simulink model "test_zynq_zcu216"  (R2018b)
settings: Solver=VariableStepAuto  StartTime=0.0  StopTime=10.0  RelTol=1e-3
undefined symbols (not defined in the file): es1
libraries: xbsIndex_r4 x19
settings Model: Creator=mcb  LastModifiedBy=mcb

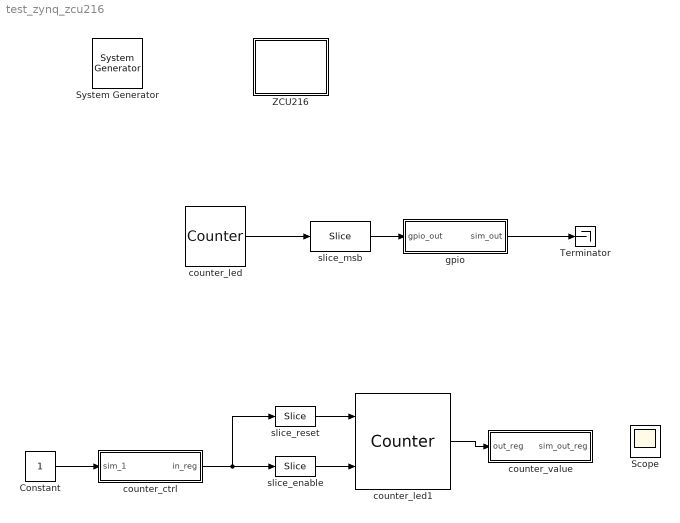
== system test_zynq_zcu216 ==
  " System Generator" : xbsIndex_r4/ System Generator  Tag=genX  xilinxfamily=zynquplusRFSOCes1  part=xczu49dr  speed=-2-e-es1  package=ffvf1760  synthesis_tool=XST  clock_wrapper=Clock Enables  directory=/home/mcb/git/casper-astro/mlib_devel/jasper_library/test_models/test_zynq_zcu216/sysgen  proj_type=Vivado  Synth_file=Vivado Synthesis Defaults  Impl_file=Vivado Implementation Defaults  testbench=off  simulink_period=1  sysclk_period=10  dcm_input_clock_period=10  incr_netlist=off  trim_vbits=Everywhere in SubSystem  dbl_ovrd=According to Block Masks  core_generation=According to Block Masks  run_coregen=off  deprecated_control=off  eval_field=0  block_type=sysgen
  Constant : Constant
  Scope : Scope
  Terminator : Terminator
  ZCU216 : Subsystem  Tag=xps:xsg  mask(xsg core config){hw_sys=ZCU216:xczu49dr, clk_src=adc_clk, clk_rate=100, sample_period=1, synthesis_tool=XST}
      mask prompts: hw_sys "Hardware Platform"; clk_src "User IP Clock source"; clk_rate "User IP Clock Rate (MHz)"; sample_period "Sample Period"; synthesis_tool "Synthesis Tool:"
      mask help:
      | The XSG Core Config block is used to configure the System Generator design
      | for the casper_xps toolflow. Settings here are used to configure the
      | Xilinx System Generator block parameters automatically, and control toolflow
      | script  execution. It needs to be at the top level of all designs being compiled
      | with the casper_xps toolflow.
      mask init:
      | xps_xsg_zcu216_conf_mask;
      mask Help: eval('xlWeb([getenv(''MLIB_ROOT''), ''\doc\html\sys_xsg_core_config\sys_xsg_core_config.html''])')
      mask TypeOptions hw_sys: ZCU216:xczu49dr
      mask TypeOptions clk_src: sys_clk | adc_clk
      mask TypeOptions synthesis_tool: Leonardo Spectrum | Synplify | Synplify Pro | XST
      mask Display: fprintf(['ZCU216']);
  counter_ctrl : Subsystem  Tag=xps:sw_reg  AncestorBlock=xps_library/Memory/software_register  mask(swreg){io_dir=From Processor, io_delay=0, init_val=0, sample_period=1, names=reg, bitwidths=32, bin_pts=0, arith_types=0, sim_port=on, show_format=off}
      mask prompts: io_dir "I/O direction"; io_delay "I/O delay"; init_val "Initial Value"; sample_period "Sample period"; names "Bitfield names [msb...lsb]"; bitwidths "Bitfield widths"; bin_pts "Bitfield binary pts"; arith_types "Bitfield types, ufix=0, fix=1, bool=2"; sim_port "Provide sim input/output?"; show_format "Print format string?"
      mask help: A 32-bit software-accessible register. Can be divided into bitfields of varying widths and types using the fields in the block mask.
      mask init:
      | swreg_init(gcb)
      settings: AttributesFormatString=1input
      mask TypeOptions io_dir: To Processor | From Processor
      mask Callback io_dir:
      | mask_enables = get_param(gcb, 'MaskEnables');
      | mask_names = get_param(gcb, 'MaskNames');
      | if strcmp(get_param(gcb, 'io_dir'), 'To Processor'),
      |     mask_enables{ismember(mask_names, 'sample_period')} = 'off';
      | else
      |     mask_enables{ismember(mask_names, 'sample_period')} = 'on';
      | end
      | set_param(gcb, 'MaskEnables', mask_enables);
      mask DialogControl ParameterTabVar0 Prompt: Setup
  counter_led : xbsIndex_r4/Counter  cnt_type=Free Running  cnt_to=Inf  operation=Up  start_count=0  cnt_by_val=1  arith_type=Unsigned  n_bits=28  bin_pt=0  load_pin=off  rst=off  en=off  explicit_period=on  period=1  use_behavioral_HDL=off  implementation=Fabric  dbl_ovrd=off  block_type=counter
  counter_led1 : xbsIndex_r4/Counter  cnt_type=Free Running  cnt_to=Inf  operation=Up  start_count=0  cnt_by_val=1  arith_type=Unsigned  n_bits=32  bin_pt=0  load_pin=off  rst=on  en=on  explicit_period=on  period=1  use_behavioral_HDL=off  implementation=Fabric  dbl_ovrd=off  block_type=counter
  counter_value : Subsystem  Tag=xps:sw_reg  AncestorBlock=xps_library/Memory/software_register  mask(swreg){io_dir=To Processor, io_delay=0, init_val=0, sample_period=1, names=reg, bitwidths=32, bin_pts=0, arith_types=0, sim_port=on, show_format=off}
      mask prompts: io_dir "I/O direction"; io_delay "I/O delay"; init_val "Initial Value"; sample_period "Sample period"; names "Bitfield names [msb...lsb]"; bitwidths "Bitfield widths"; bin_pts "Bitfield binary pts"; arith_types "Bitfield types, ufix=0, fix=1, bool=2"; sim_port "Provide sim input/output?"; show_format "Print format string?"
      mask help: A 32-bit software-accessible register. Can be divided into bitfields of varying widths and types using the fields in the block mask.
      mask init:
      | swreg_init(gcb)
      settings: AttributesFormatString=1output
      mask TypeOptions io_dir: To Processor | From Processor
      mask Callback io_dir:
      | mask_enables = get_param(gcb, 'MaskEnables');
      | mask_names = get_param(gcb, 'MaskNames');
      | if strcmp(get_param(gcb, 'io_dir'), 'To Processor'),
      |     mask_enables{ismember(mask_names, 'sample_period')} = 'off';
      | else
      |     mask_enables{ismember(mask_names, 'sample_period')} = 'on';
      | end
      | set_param(gcb, 'MaskEnables', mask_enables);
      mask DialogControl ParameterTabVar0 Prompt: Setup
  gpio : Subsystem  Tag=xps:gpio  AncestorBlock=xps_library/IO/gpio  mask(gpio){io_group_params_forwarded=on, io_group=ROACH2:led, io_group_real=led, io_group_custom=0, io_dir=out, arith_type=Boolean, bitwidth=1, bin_pt=0, bit_index=0, sample_period=1, use_single_ended=off, use_ddr=off, reg_iob=on, reg_clk_phase=0, termination=None}
      mask prompts: io_group_params_forwarded "Have the io_group params been forwarded yet?"; io_group "I/O group"; io_group_real "I/O group"; io_group_custom "Custom I/O group"; io_dir "I/O direction"; arith_type "Data Type"; bitwidth "Data bitwidth"; bin_pt "Data binary point"; bit_index "GPIO bit index"; sample_period "Sample period"; use_single_ended "Use as single-ended"; use_ddr "Use DDR"; reg_iob "Pack register in the pad"; reg_clk_phase "Register clock phase"; termination "Termination method"
      mask help:
      | GPIO interfaces for CASPER hardware.
      |
      | For usage of LEDs on SKARAB boards, please note that the board will boot into 'BSP mode' by default. To change the control of the Front Panel LEDs to your design, execute the command 'control_front_panel_leds_write()' on your SKARAB CASPERFPGA object via the transport layer.
      |
      | For more information please click help below.
      mask init:
      | gpio_mask;
      mask Help: If you've come here for more help, unfortunately I'm going to direct you to the ska-sa/casperfpga wiki. The documentation at https://github.com/ska-sa/casperfpga/wiki/SKARAB-Front-Panel-LED-Manager outlines the signals that are used to control the SKARAB's Front Panel LEDs by default, and the mechanism by which you can switch control to the DSP Design.
      mask TypeOptions io_group: ROACH:aux0_clk | ROACH:aux1_clk | ROACH:led | ROACH:gpioa | ROACH:gpioa_oe_n | ROACH:gpiob | ROACH:gpiob_oe_n | ROACH:qsh | ROACH:zdok0 | ROACH:zdok1 | ROACH2:aux_clk | ROACH2:led | ROACH2:gpio | ROACH2:qsh | ROACH2:sync_in | ROACH2:sync_out | ROACH2:zdok0 | ROACH2:zdok1 | custom:custom
      mask TypeOptions io_group_real: led | gpio | sync_in | sync_out | zdok0 | zdok1 | aux_clk_diff | custom
      mask Callback io_group_real:
      | if ~isempty(find(strcmp(get_param(gcb, 'io_group_real'), {'zdok0' 'zdok1' 'sync_in' 'sync_out'})))
      |     set_param(gcb, 'MaskEnables', {'off', 'off', 'on','off','on','on','on','on','on','on','on','on','on','on','on'});
      | elseif ~isempty(find(strcmp(get_param(gcb, 'io_group_real'), {'custom'})))
      |     set_param(gcb, 'MaskEnables', {'off', 'off', 'on','on','on','on','on','on','on','on','off','on','on','on','on'});
      | else
      |     set_param(gcb, 'MaskEnables', {'off', 'off', 'on','off','on','on','on','on','on','on','off','on','on','on','on'});
      | end
      mask TypeOptions io_dir: in | out
      mask Callback io_dir:
      | if ~isempty(find(strcmp(get_param(gcb, 'io_group_real'), {'zdok0' 'zdok1' 'sync_in' 'sync_out'})))
      |     set_param(gcb, 'MaskVisibilities', {'off', 'off','on','on','on','on','on','on','on','on','on','on','on','on','on'});
      | else
      |     set_param(gcb, 'MaskVisibilities', {'off', 'off','on','on','on','on','on','on','on','on','off','on','on','on','on'});
      | end
      mask TypeOptions arith_type: Boolean | Unsigned | Signed  (2's comp)
      mask Callback use_ddr:
      | if strcmp(get_param(gcb,'use_ddr'),'on')
      |     set_param(gcb,'reg_iob','on');
      |     set_param(gcb,'MaskEnables', {'off' 'off' 'on' 'on' 'on' 'on' 'on' 'on' 'on' 'on' 'on' 'on' 'off' 'on' 'on'});
      | else
      |     set_param(gcb,'MaskEnables', {'off' 'off' 'on' 'on' 'on' 'on' 'on' 'on' 'on' 'on' 'on' 'on' 'on' 'on' 'on'});
      | end
      mask TypeOptions reg_clk_phase: 0 | 90 | 180 | 270
      mask TypeOptions termination: None | Pullup | Pulldown
  slice_enable : xbsIndex_r4/Slice  nbits=1  boolean_output=on  mode=Lower Bit Location + Width  bit1=0  base1=MSB of Input  bit0=0  base0=LSB of Input  dbl_ovrd=off  block_type=slice
  slice_msb : xbsIndex_r4/Slice  nbits=1  boolean_output=off  mode=Upper Bit Location + Width  bit1=0  base1=MSB of Input  bit0=0  base0=LSB of Input  dbl_ovrd=off  block_type=slice
  slice_reset : xbsIndex_r4/Slice  nbits=1  boolean_output=on  mode=Lower Bit Location + Width  bit1=0  base1=MSB of Input  bit0=1  base0=LSB of Input  dbl_ovrd=off  block_type=slice
  wires:
  gpio/1(sim_out) -> Terminator/1
  slice_msb/1 -> gpio/1(gpio_out)
  counter_led/1 -> slice_msb/1
  counter_ctrl/1(in_reg) -> slice_reset/1, slice_enable/1
  Constant/1 -> counter_ctrl/1(sim_1)
  counter_led1/1 -> counter_value/1(out_reg)
  slice_enable/1 -> counter_led1/2
  slice_reset/1 -> counter_led1/1
  ? -> Scope/1

== system test_zynq_zcu216/ZCU216 ==

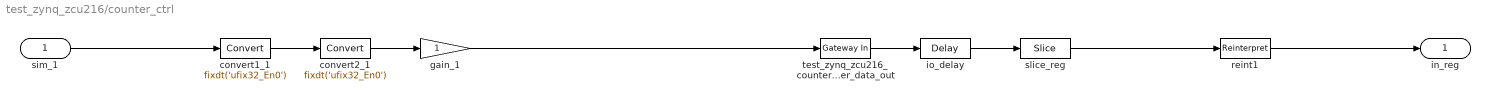
== system test_zynq_zcu216/counter_ctrl ==
  sim_1 : Inport
  convert1_1 : DataTypeConversion  OutDataTypeStr=fixdt('ufix32_En0')  LockScale=on
  convert2_1 : DataTypeConversion  OutDataTypeStr=fixdt('ufix32_En0')  ConvertRealWorld=Stored Integer (SI)  LockScale=on
  gain_1 : Gain
  io_delay : xbsIndex_r4/Delay  rst=off  infoeditControl=Selection of Reset will increase slice count due to use of real FFs and instead of SRLs  en=off  latency=0  reg_retiming=on  dbl_ovrd=off  block_type=delay
  reint1 : xbsIndex_r4/Reinterpret  force_arith_type=on  arith_type=Unsigned  force_bin_pt=on  bin_pt=0  block_type=reinterpret
  slice_reg : xbsIndex_r4/Slice  nbits=32  boolean_output=off  mode=Lower Bit Location + Width  bit1=0  base1=MSB of Input  bit0=0  base0=LSB of Input  dbl_ovrd=off  block_type=slice
  test_zynq_zcu216_counter_ctrl_user_data_out : xbsIndex_r4/Gateway In  gui_display_data_type=Fixed-point  arith_type=Unsigned  n_bits=32  bin_pt=0  preci_type=Single  exp_width=8  frac_width=24  rows=1  columns=1  quantization="Round  (unbiased: +/- Inf)"  overflow=Saturate  period=1  UseAsADC=off  ADCChannel='1'  interface=None  automatic_assignment=on  address_offset=hex2dec('00')  intf_name=''  intf_description=''  default_value=0  timing_constraint=None  locs_specified=off  LOCs={}  io_standard={}  inherit_from_input=off  hdl_port=on  dbl_ovrd=off  block_type=gatewayin
  in_reg : Outport
  wires:
  test_zynq_zcu216_counter_ctrl_user_data_out/1 -> io_delay/1
  sim_1/1 -> convert1_1/1
  convert1_1/1 -> convert2_1/1
  convert2_1/1 -> gain_1/1
  gain_1/1 -> test_zynq_zcu216_counter_ctrl_user_data_out/1
  io_delay/1 -> slice_reg/1
  slice_reg/1 -> reint1/1
  reint1/1 -> in_reg/1

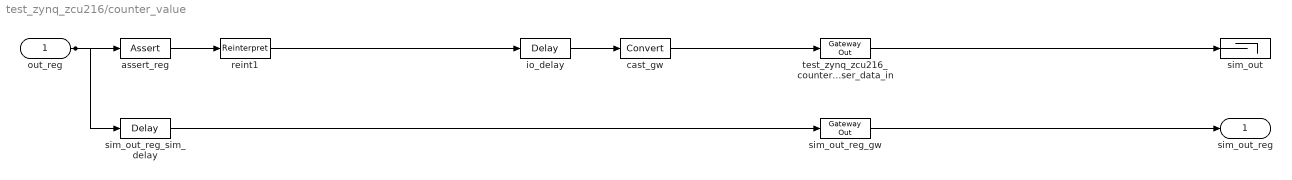
== system test_zynq_zcu216/counter_value ==
  out_reg : Inport
  assert_reg : xbsIndex_r4/Assert  assert_type=on  type_source=Explicitly  gui_display_data_type=Fixed-point  arith_type=Unsigned  n_bits=32  bin_pt=0  preci_type=Single  exp_width=8  frac_width=24  assert_rate=off  rate_source=Explicitly  period=1  output_port=on  block_type=assert
  cast_gw : xbsIndex_r4/Convert  gui_display_data_type=Fixed-point  arith_type=Unsigned  n_bits=32  bin_pt=0  float_type=Single  exp_bits=8  fraction_bits=24  quantization=Truncate  overflow=Wrap  en=off  latency=1  pipeline=off  dbl_ovrd=off  block_type=convert
  io_delay : xbsIndex_r4/Delay  rst=off  infoeditControl=Selection of Reset will increase slice count due to use of real FFs and instead of SRLs  en=off  latency=0  reg_retiming=on  dbl_ovrd=off  block_type=delay
  reint1 : xbsIndex_r4/Reinterpret  force_arith_type=on  arith_type=Unsigned  force_bin_pt=on  bin_pt=0  block_type=reinterpret
  sim_out : Terminator
  sim_out_reg_gw : xbsIndex_r4/Gateway Out  inherit_from_input=off  hdl_port=off  rows=1  columns=1  UseAsDAC=off  DACChannel='1'  interface=None  automatic_assignment=on  address_offset=hex2dec('00')  intf_name=''  intf_description=''  timing_constraint=None  locs_specified=off  LOCs={}  io_standard={}  block_type=gatewayout
  sim_out_reg_sim_delay : xbsIndex_r4/Delay  rst=off  infoeditControl=Selection of Reset will increase slice count due to use of real FFs and instead of SRLs  en=off  latency=1  reg_retiming=on  dbl_ovrd=off  block_type=delay
  test_zynq_zcu216_counter_value_user_data_in : xbsIndex_r4/Gateway Out  inherit_from_input=off  hdl_port=on  rows=1  columns=1  UseAsDAC=off  DACChannel='1'  interface=None  automatic_assignment=on  address_offset=hex2dec('00')  intf_name=''  intf_description=''  timing_constraint=None  locs_specified=off  LOCs={}  io_standard={}  block_type=gatewayout
  sim_out_reg : Outport
  wires:
  sim_out_reg_sim_delay/1 -> sim_out_reg_gw/1
  sim_out_reg_gw/1 -> sim_out_reg/1
  io_delay/1 -> cast_gw/1
  cast_gw/1 -> test_zynq_zcu216_counter_value_user_data_in/1
  test_zynq_zcu216_counter_value_user_data_in/1 -> sim_out/1
  out_reg/1 -> sim_out_reg_sim_delay/1, assert_reg/1
  assert_reg/1 -> reint1/1
  reint1/1 -> io_delay/1

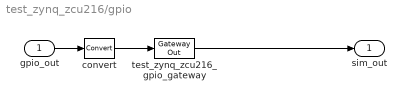
== system test_zynq_zcu216/gpio ==
  gpio_out : Inport
  convert : xbsIndex_r4/Convert  gui_display_data_type=Fixed-point  arith_type=Boolean  n_bits=1  bin_pt=0  float_type=Single  exp_bits=8  fraction_bits=24  quantization=Truncate  overflow=Wrap  en=off  latency=1  pipeline=off  dbl_ovrd=off  block_type=convert
  test_zynq_zcu216_gpio_gateway : xbsIndex_r4/Gateway Out  inherit_from_input=off  hdl_port=on  rows=1  columns=1  UseAsDAC=off  DACChannel='1'  interface=None  automatic_assignment=on  address_offset=hex2dec('00')  intf_name=''  intf_description=''  timing_constraint=None  locs_specified=off  LOCs={}  io_standard={}  block_type=gatewayout
  sim_out : Outport
  wires:
  gpio_out/1 -> convert/1
  convert/1 -> test_zynq_zcu216_gpio_gateway/1
  test_zynq_zcu216_gpio_gateway/1 -> sim_out/1
